simulink model "DUALportRAMinterface_test"  (R2024a)
settings: Solver=FixedStepDiscrete  StartTime=0.0  StopTime=1100  RelTol=1e-3
values from neighbouring files (symbols this model uses):
  Ts = 1/Fs    (= 7.50007500075e-06)    [new_generation_coeff.m]    (also in simon_test.m; simple_fft_test.m = 1/F; testPSD_c2d.m; testPSD_simulink.m)
libraries: hdlsllib x34, simulink x1
settings Model: DataTypeOverride=Off  SimulationMode=rapid-accelerator  Creator=Simon  LastModifiedBy=Simon
settings OptimizationCC: BlockReduction=off  ConditionallyExecuteInputs=off  DefaultParameterBehavior=Inlined  InheritOutputTypeSmallerThanSingle=on
settings DebuggingCC: AlgebraicLoopMsg=error  SingleTaskRateTransMsg=error  UnconnectedInputMsg=warning  UnconnectedOutputMsg=warning  UnconnectedLineMsg=warning
settings HardwareCC: ProdBitPerPointer=32  ProdBitPerSizeT=32  ProdBitPerPtrDiffT=32  ProdLargestAtomicFloat=None  ProdIntDivRoundTo=Undefined  ProdEndianess=Unspecified  ProdWordSize=32  ProdHWDeviceType=ASIC/FPGA->ASIC/FPGA  TargetBitPerPointer=64  TargetBitPerSizeT=64  TargetBitPerPtrDiffT=64  TargetLongLongMode=on  TargetIntDivRoundTo=Zero  TargetEndianess=LittleEndian  TargetWordSize=64  TargetHWDeviceType=Custom Processor->MATLAB Host Computer  ProdEqTarget=off

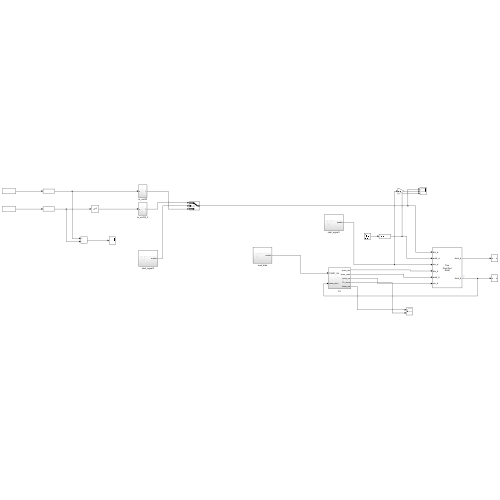
[thumbnail: Simulink's stored preview of the top-level diagram]
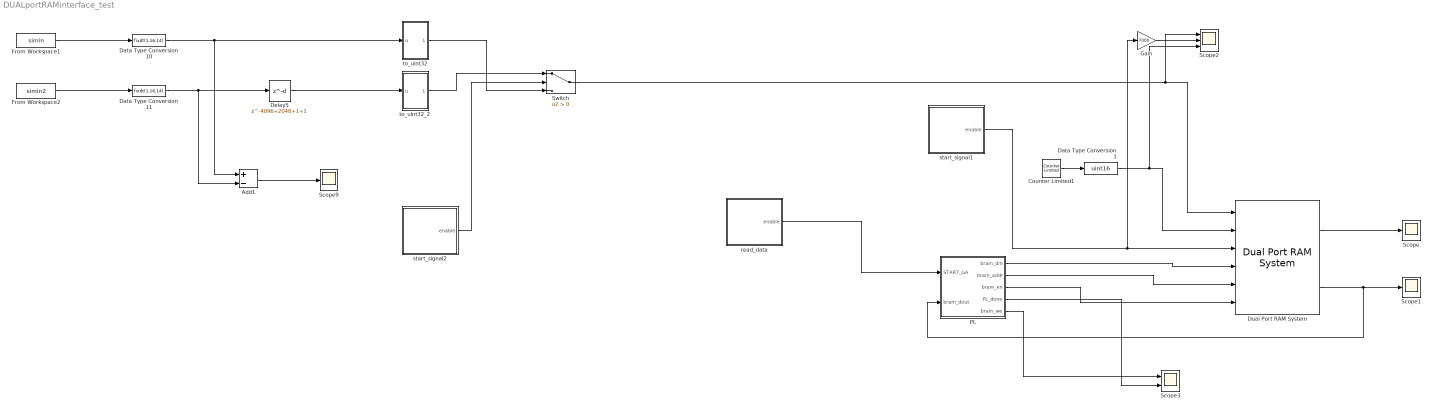
== system DUALportRAMinterface_test ==
  Add1 : Sum  Inputs=+-
  Counter Limited1 : simulink/Sources/Counter Limited  uplimit=14000  tsamp=Ts
  Data Type Conversion1 : DataTypeConversion  OutDataTypeStr=uint16  SaturateOnIntegerOverflow=off  RndMeth=Floor
  Data Type Conversion10 : DataTypeConversion  OutDataTypeStr=fixdt(1,16,14)  SaturateOnIntegerOverflow=off  RndMeth=Floor
  Data Type Conversion11 : DataTypeConversion  OutDataTypeStr=fixdt(1,16,14)  SaturateOnIntegerOverflow=off  RndMeth=Floor
  Delay5 : Delay  DelayLength=4096+2048+1+1  InitialCondition=0  SampleTime=Ts
  Dual Port RAM System : hdlsllib/HDL RAMs/Dual Port RAM System  RAMType=True dual port  AsyncRead=off  WriteOutputValue=New data  RAMInitialValue=0  allowBusInputs=off  WritesHaveOutput=on  NumReads=0  NumWrites=1  SimulateUsing=Code generation
  From Workspace1 : FromWorkspace  VariableName=simin  SampleTime=Ts
  From Workspace2 : FromWorkspace  VariableName=simin2  SampleTime=Ts
  Gain : Gain  Gain=7000
  PL : Subsystem
  Scope : Scope
  Scope1 : Scope
  Scope2 : Scope  NumInputPorts=3
  Scope3 : Scope  NumInputPorts=2
  Scope9 : Scope
  Switch : Switch  Criteria=u2 > Threshold  SaturateOnIntegerOverflow=off  InputSameDT=off  OutDataTypeStr=Inherit: Same as first input
  read_data : Subsystem
  start_signal1 : Subsystem
  start_signal2 : Subsystem
  to_uint32 : Subsystem
  to_uint32_2 : Subsystem
  wires:
  Dual Port RAM System/1 -> Scope/1
  Counter Limited1/1 -> Data Type Conversion1/1
  Data Type Conversion1/1 -> Scope2/3, Dual Port RAM System/2
  start_signal1/1(enable) -> Dual Port RAM System/3, Gain/1
  PL/1(bram_din) -> Dual Port RAM System/4
  PL/2(bram_addr) -> Dual Port RAM System/5
  PL/3(bram_en) -> Dual Port RAM System/6
  Gain/1 -> Scope2/2
  read_data/1(enable) -> PL/1(START_GA)
  Dual Port RAM System/2 -> Scope1/1, PL/2(bram_dout)
  From Workspace1/1 -> Data Type Conversion10/1
  From Workspace2/1 -> Data Type Conversion11/1
  to_uint32/1(Out1) -> Switch/3
  to_uint32_2/1(Out1) -> Switch/1
  start_signal2/1(enable) -> Switch/2
  Delay5/1 -> to_uint32_2/1(u)
  Switch/1 -> Scope2/1, Dual Port RAM System/1
  Data Type Conversion11/1 -> Delay5/1, Add1/2
  Add1/1 -> Scope9/1
  Data Type Conversion10/1 -> Add1/1, to_uint32/1(u)
  PL/4(PL_done) -> Scope3/2
  PL/5(bram_we) -> Scope3/1

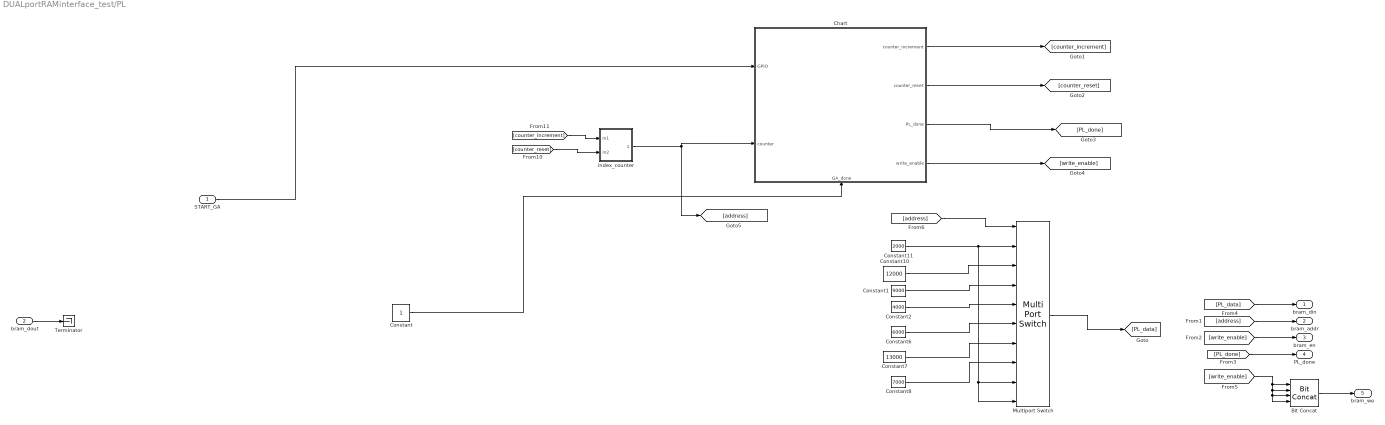
== system DUALportRAMinterface_test/PL ==
  START_GA : Inport
  bram_dout : Inport  Port=2
  Bit Concat : hdlsllib/Logic and Bit Operations/Bit Concat  numInputs=4
  Chart : Stateflow chart  TreatAsAtomicUnit=on
      settings: PortSchema="{\"entries\":[{\"content\":{\"sides\":[{\"content\":{\"connectorIds\":[\"In2\",\"In3\"]},\"type\":\"ConnectorPlacement.EquallySpacedRectSide\",\"uuid\":\"f3ce331f-c708-4668-a9cb-fb327ea74ab5\"},{\"content\":{\"connectorIds\":[\"Out1\",\"Out2\",\"Out3\",\"Out4\"],\"side\":\"RIGHT\"},\"type\":\"ConnectorPlacement.EquallySpacedRectSide\",\"uuid\":\"3766927a-abff-497d-9544-2098881ba174\"},{\"content\":{\"side\":\"TOP\"},\"type\":\"ConnectorPlacement.EquallySpacedRectSide\",\"uuid\":\"ebfe3d64-ee7d-4953-a6ba-e7e40988decf\"},{\"content\":{\"connectorIds\":[\"In1\"],\"side\":\"BOTTOM\"},\"type\":\"ConnectorPlacement.EquallySpacedRectSide\",\"uuid\":\"f39ceaf8-4df7-4e40-9de5-da7597831fb4\"}]},\"type\":\"ConnectorPlacement.EquallySpacedConnector\",\"uuid\":\"89f60450-5933-42bb-b72b-5f8ec55483e0\"}],\"packageUris\":[\"http://schema.mathworks.com/mf0/Connector/R2020b\"],\"version\":\"1.0\"}"
  Constant : Constant  OutDataTypeStr=boolean
  Constant1 : Constant  Value=9000  OutDataTypeStr=uint32  SampleTime=Ts
  Constant10 : Constant  Value=12000  OutDataTypeStr=uint32  SampleTime=Ts
  Constant11 : Constant  Value=2000  OutDataTypeStr=uint32  SampleTime=Ts
  Constant2 : Constant  Value=4000  OutDataTypeStr=uint32  SampleTime=Ts
  Constant6 : Constant  Value=6000  OutDataTypeStr=uint32  SampleTime=Ts
  Constant7 : Constant  Value=13000  OutDataTypeStr=uint32  SampleTime=Ts
  Constant8 : Constant  Value=7000  OutDataTypeStr=uint32  SampleTime=Ts
  Multiport Switch : MultiPortSwitch  DataPortOrder=Specify indices  Inputs=8  DataPortIndices={0,1,2,3,4,5,6,7}  DataPortForDefault=Additional data port  DiagnosticForDefault=None  SaturateOnIntegerOverflow=off  InputSameDT=off
  Terminator : Terminator
  index_counter : Subsystem
  bram_din : Outport
  bram_addr : Outport  Port=2
  bram_en : Outport  Port=3
  PL_done : Outport  Port=4
  bram_we : Outport  Port=5
  wires:
  Multiport Switch/1 -> [PL_data]
  [counter_reset] -> index_counter/2(In2)
  index_counter/1(index_counter) -> Chart/3(counter), [address]
  [address] -> bram_addr/1
  [counter_increment] -> index_counter/1(In1)
  [address] -> Multiport Switch/1
  Chart/4(write_enable) -> [write_enable]
  Constant/1 -> Chart/1(GA_done)
  START_GA/1 -> Chart/2(GPIO)
  Chart/2(counter_reset) -> [counter_reset]
  Chart/1(counter_increment) -> [counter_increment]
  [PL_data] -> bram_din/1
  [write_enable] -> bram_en/1
  Constant11/1 -> Multiport Switch/10, Multiport Switch/9, Multiport Switch/2
  Constant10/1 -> Multiport Switch/3
  Constant1/1 -> Multiport Switch/4
  Constant2/1 -> Multiport Switch/5
  Constant6/1 -> Multiport Switch/6
  Constant7/1 -> Multiport Switch/7
  Constant8/1 -> Multiport Switch/8
  bram_dout/1 -> Terminator/1
  [PL_done] -> PL_done/1
  Chart/3(PL_done) -> [PL_done]
  [write_enable] -> Bit Concat/4, Bit Concat/3, Bit Concat/2, Bit Concat/1
  Bit Concat/1 -> bram_we/1

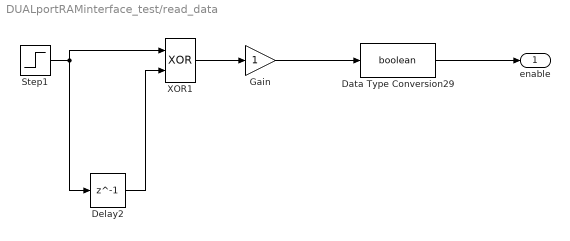
== system DUALportRAMinterface_test/read_data ==
  Data Type Conversion29 : DataTypeConversion  OutDataTypeStr=boolean  SaturateOnIntegerOverflow=off  RndMeth=Floor
  Delay2 : Delay  DelayLength=1  InitialCondition=0  SampleTime=Ts
  Gain : Gain
  Step1 : Step  Time=Ts*14000  SampleTime=Ts
  XOR1 : Logic  Operator=XOR  IconShape=distinctive  AllPortsSameDT=off  OutDataTypeStr=boolean
  enable : Outport
  wires:
  XOR1/1 -> Gain/1
  Step1/1 -> Delay2/1, XOR1/1
  Delay2/1 -> XOR1/2
  Gain/1 -> Data Type Conversion29/1
  Data Type Conversion29/1 -> enable/1

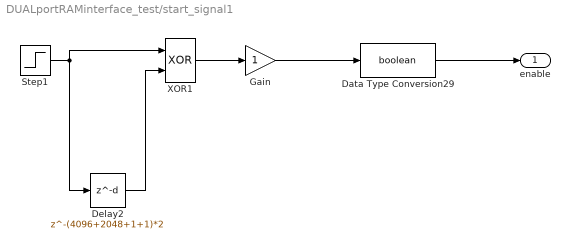
== system DUALportRAMinterface_test/start_signal1 ==
  Data Type Conversion29 : DataTypeConversion  OutDataTypeStr=boolean  SaturateOnIntegerOverflow=off  RndMeth=Floor
  Delay2 : Delay  DelayLength=(4096+2048+1+1)*2  InitialCondition=0  SampleTime=Ts
  Gain : Gain
  Step1 : Step  Time=Ts*0  SampleTime=Ts
  XOR1 : Logic  Operator=XOR  IconShape=distinctive  AllPortsSameDT=off  OutDataTypeStr=boolean
  enable : Outport
  wires:
  Data Type Conversion29/1 -> enable/1
  Gain/1 -> Data Type Conversion29/1
  Delay2/1 -> XOR1/2
  Step1/1 -> XOR1/1, Delay2/1
  XOR1/1 -> Gain/1

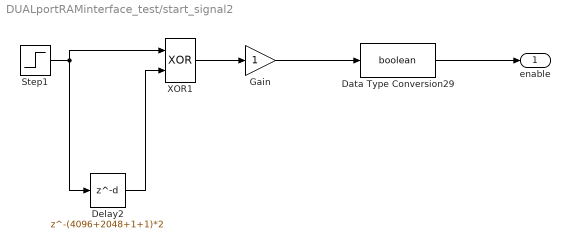
== system DUALportRAMinterface_test/start_signal2 ==
  Data Type Conversion29 : DataTypeConversion  OutDataTypeStr=boolean  SaturateOnIntegerOverflow=off  RndMeth=Floor
  Delay2 : Delay  DelayLength=(4096+2048+1+1)*2  InitialCondition=0  SampleTime=Ts
  Gain : Gain
  Step1 : Step  Time=Ts*(4096+2048+1+1)  SampleTime=Ts
  XOR1 : Logic  Operator=XOR  IconShape=distinctive  AllPortsSameDT=off  OutDataTypeStr=boolean
  enable : Outport
  wires:
  XOR1/1 -> Gain/1
  Step1/1 -> Delay2/1, XOR1/1
  Delay2/1 -> XOR1/2
  Gain/1 -> Data Type Conversion29/1
  Data Type Conversion29/1 -> enable/1

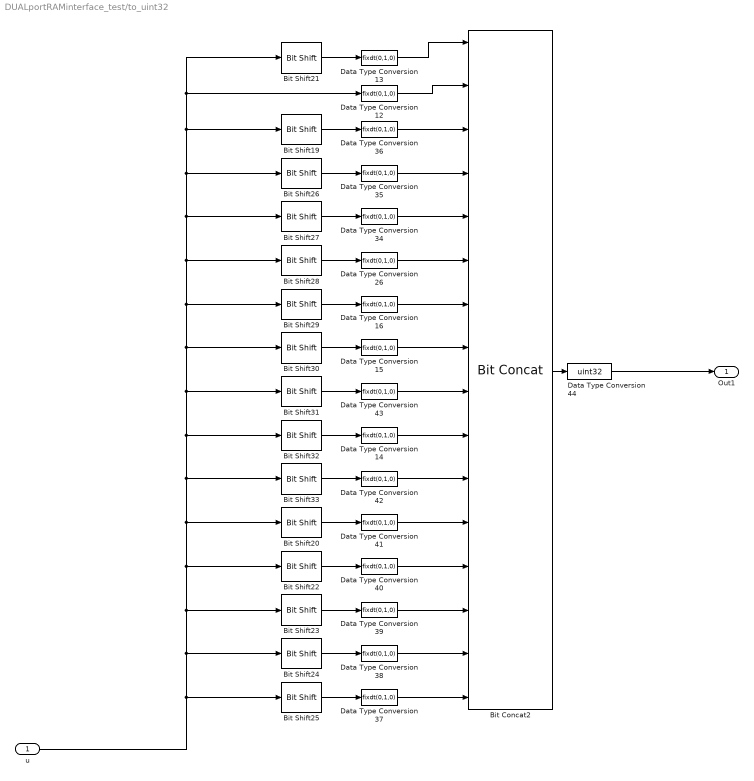
== system DUALportRAMinterface_test/to_uint32 ==
  u : Inport
  Bit Concat2 : hdlsllib/Logic and Bit Operations/Bit Concat  numInputs=16
  Bit Shift19 : hdlsllib/Logic and Bit Operations/Bit Shift  mode=Shift Left Logical  N=1
  Bit Shift20 : hdlsllib/Logic and Bit Operations/Bit Shift  mode=Shift Left Logical  N=10
  Bit Shift21 : hdlsllib/Logic and Bit Operations/Bit Shift  mode=Shift Right Logical  N=1
  Bit Shift22 : hdlsllib/Logic and Bit Operations/Bit Shift  mode=Shift Left Logical  N=11
  Bit Shift23 : hdlsllib/Logic and Bit Operations/Bit Shift  mode=Shift Left Logical  N=12
  Bit Shift24 : hdlsllib/Logic and Bit Operations/Bit Shift  mode=Shift Left Logical  N=13
  Bit Shift25 : hdlsllib/Logic and Bit Operations/Bit Shift  mode=Shift Left Logical  N=14
  Bit Shift26 : hdlsllib/Logic and Bit Operations/Bit Shift  mode=Shift Left Logical  N=2
  Bit Shift27 : hdlsllib/Logic and Bit Operations/Bit Shift  mode=Shift Left Logical  N=3
  Bit Shift28 : hdlsllib/Logic and Bit Operations/Bit Shift  mode=Shift Left Logical  N=4
  Bit Shift29 : hdlsllib/Logic and Bit Operations/Bit Shift  mode=Shift Left Logical  N=5
  Bit Shift30 : hdlsllib/Logic and Bit Operations/Bit Shift  mode=Shift Left Logical  N=6
  Bit Shift31 : hdlsllib/Logic and Bit Operations/Bit Shift  mode=Shift Left Logical  N=7
  Bit Shift32 : hdlsllib/Logic and Bit Operations/Bit Shift  mode=Shift Left Logical  N=8
  Bit Shift33 : hdlsllib/Logic and Bit Operations/Bit Shift  mode=Shift Left Logical  N=9
  Data Type Conversion{12..16,26,34..43} (16 alike) : DataTypeConversion  OutDataTypeStr=fixdt(0,1,0)  SaturateOnIntegerOverflow=off  RndMeth=Floor
  Data Type Conversion44 : DataTypeConversion  OutDataTypeStr=uint32  SaturateOnIntegerOverflow=off  RndMeth=Floor
  Out1 : Outport
  wires:
  Bit Shift22/1 -> Data Type Conversion40/1
  Bit Shift27/1 -> Data Type Conversion34/1
  Data Type Conversion36/1 -> Bit Concat2/3
  u/1 -> Bit Shift21/1, Data Type Conversion12/1, Bit Shift19/1, Bit Shift26/1, Bit Shift27/1, Bit Shift28/1, Bit Shift29/1, Bit Shift30/1, Bit Shift31/1, Bit Shift32/1, Bit Shift33/1, Bit Shift20/1, Bit Shift22/1, Bit Shift23/1, Bit Shift24/1, Bit Shift25/1
  Bit Shift20/1 -> Data Type Conversion41/1
  Data Type Conversion13/1 -> Bit Concat2/1
  Data Type Conversion40/1 -> Bit Concat2/13
  Bit Shift31/1 -> Data Type Conversion43/1
  Data Type Conversion26/1 -> Bit Concat2/6
  Data Type Conversion44/1 -> Out1/1
  Data Type Conversion35/1 -> Bit Concat2/4
  Data Type Conversion42/1 -> Bit Concat2/11
  Bit Shift19/1 -> Data Type Conversion36/1
  Data Type Conversion38/1 -> Bit Concat2/15
  Bit Shift25/1 -> Data Type Conversion37/1
  Data Type Conversion15/1 -> Bit Concat2/8
  Bit Shift30/1 -> Data Type Conversion15/1
  Data Type Conversion12/1 -> Bit Concat2/2
  Bit Shift32/1 -> Data Type Conversion14/1
  Data Type Conversion39/1 -> Bit Concat2/14
  Data Type Conversion34/1 -> Bit Concat2/5
  Data Type Conversion43/1 -> Bit Concat2/9
  Data Type Conversion16/1 -> Bit Concat2/7
  Bit Shift33/1 -> Data Type Conversion42/1
  Bit Shift24/1 -> Data Type Conversion38/1
  Data Type Conversion41/1 -> Bit Concat2/12
  Bit Shift23/1 -> Data Type Conversion39/1
  Bit Shift29/1 -> Data Type Conversion16/1
  Data Type Conversion37/1 -> Bit Concat2/16
  Bit Shift28/1 -> Data Type Conversion26/1
  Bit Shift21/1 -> Data Type Conversion13/1
  Bit Shift26/1 -> Data Type Conversion35/1
  Bit Concat2/1 -> Data Type Conversion44/1
  Data Type Conversion14/1 -> Bit Concat2/10

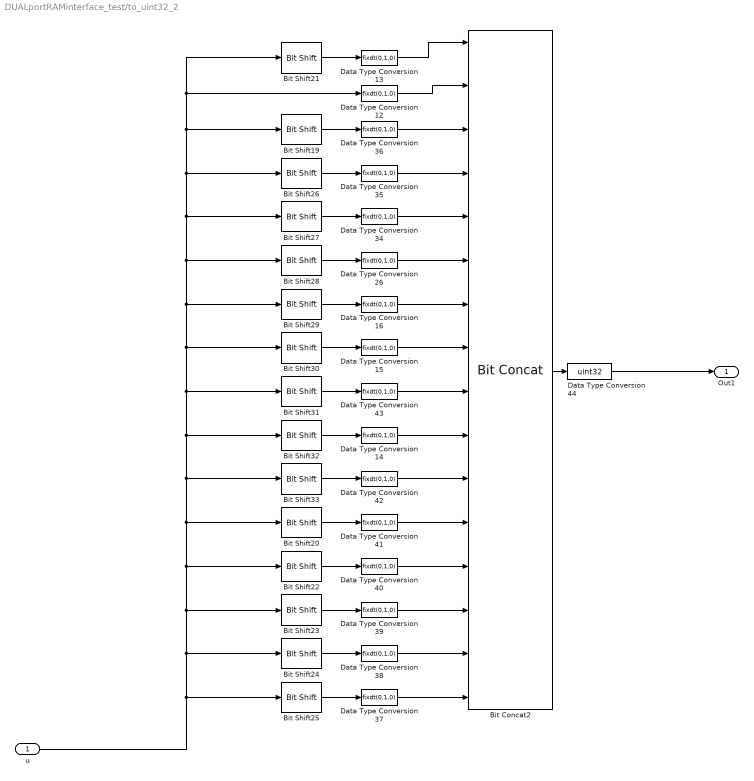
== system DUALportRAMinterface_test/to_uint32_2 ==
  u : Inport
  Bit Concat2 : hdlsllib/Logic and Bit Operations/Bit Concat  numInputs=16
  Bit Shift19 : hdlsllib/Logic and Bit Operations/Bit Shift  mode=Shift Left Logical  N=1
  Bit Shift20 : hdlsllib/Logic and Bit Operations/Bit Shift  mode=Shift Left Logical  N=10
  Bit Shift21 : hdlsllib/Logic and Bit Operations/Bit Shift  mode=Shift Right Logical  N=1
  Bit Shift22 : hdlsllib/Logic and Bit Operations/Bit Shift  mode=Shift Left Logical  N=11
  Bit Shift23 : hdlsllib/Logic and Bit Operations/Bit Shift  mode=Shift Left Logical  N=12
  Bit Shift24 : hdlsllib/Logic and Bit Operations/Bit Shift  mode=Shift Left Logical  N=13
  Bit Shift25 : hdlsllib/Logic and Bit Operations/Bit Shift  mode=Shift Left Logical  N=14
  Bit Shift26 : hdlsllib/Logic and Bit Operations/Bit Shift  mode=Shift Left Logical  N=2
  Bit Shift27 : hdlsllib/Logic and Bit Operations/Bit Shift  mode=Shift Left Logical  N=3
  Bit Shift28 : hdlsllib/Logic and Bit Operations/Bit Shift  mode=Shift Left Logical  N=4
  Bit Shift29 : hdlsllib/Logic and Bit Operations/Bit Shift  mode=Shift Left Logical  N=5
  Bit Shift30 : hdlsllib/Logic and Bit Operations/Bit Shift  mode=Shift Left Logical  N=6
  Bit Shift31 : hdlsllib/Logic and Bit Operations/Bit Shift  mode=Shift Left Logical  N=7
  Bit Shift32 : hdlsllib/Logic and Bit Operations/Bit Shift  mode=Shift Left Logical  N=8
  Bit Shift33 : hdlsllib/Logic and Bit Operations/Bit Shift  mode=Shift Left Logical  N=9
  Data Type Conversion{12..16,26,34..43} (16 alike) : DataTypeConversion  OutDataTypeStr=fixdt(0,1,0)  SaturateOnIntegerOverflow=off  RndMeth=Floor
  Data Type Conversion44 : DataTypeConversion  OutDataTypeStr=uint32  SaturateOnIntegerOverflow=off  RndMeth=Floor
  Out1 : Outport
  wires:
  Data Type Conversion14/1 -> Bit Concat2/10
  Bit Concat2/1 -> Data Type Conversion44/1
  Bit Shift26/1 -> Data Type Conversion35/1
  Bit Shift21/1 -> Data Type Conversion13/1
  Bit Shift28/1 -> Data Type Conversion26/1
  Data Type Conversion37/1 -> Bit Concat2/16
  Bit Shift29/1 -> Data Type Conversion16/1
  Bit Shift23/1 -> Data Type Conversion39/1
  Data Type Conversion41/1 -> Bit Concat2/12
  Bit Shift24/1 -> Data Type Conversion38/1
  Bit Shift33/1 -> Data Type Conversion42/1
  Data Type Conversion16/1 -> Bit Concat2/7
  Data Type Conversion43/1 -> Bit Concat2/9
  Data Type Conversion34/1 -> Bit Concat2/5
  Data Type Conversion39/1 -> Bit Concat2/14
  Bit Shift32/1 -> Data Type Conversion14/1
  Data Type Conversion12/1 -> Bit Concat2/2
  Bit Shift30/1 -> Data Type Conversion15/1
  Data Type Conversion15/1 -> Bit Concat2/8
  Bit Shift25/1 -> Data Type Conversion37/1
  Data Type Conversion38/1 -> Bit Concat2/15
  Bit Shift19/1 -> Data Type Conversion36/1
  Data Type Conversion42/1 -> Bit Concat2/11
  Data Type Conversion35/1 -> Bit Concat2/4
  Data Type Conversion44/1 -> Out1/1
  Data Type Conversion26/1 -> Bit Concat2/6
  Bit Shift31/1 -> Data Type Conversion43/1
  Data Type Conversion40/1 -> Bit Concat2/13
  Data Type Conversion13/1 -> Bit Concat2/1
  Bit Shift20/1 -> Data Type Conversion41/1
  u/1 -> Bit Shift25/1, Bit Shift24/1, Bit Shift23/1, Bit Shift22/1, Bit Shift20/1, Bit Shift33/1, Bit Shift32/1, Bit Shift31/1, Bit Shift30/1, Bit Shift29/1, Bit Shift28/1, Bit Shift27/1, Bit Shift26/1, Bit Shift19/1, Data Type Conversion12/1, Bit Shift21/1
  Data Type Conversion36/1 -> Bit Concat2/3
  Bit Shift27/1 -> Data Type Conversion34/1
  Bit Shift22/1 -> Data Type Conversion40/1

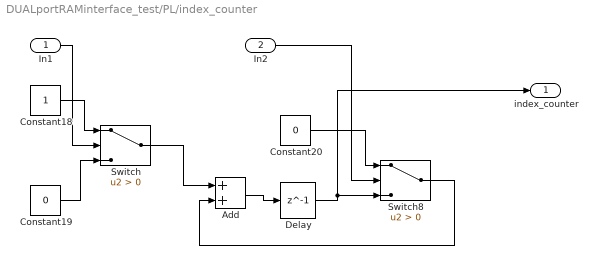
== system DUALportRAMinterface_test/PL/index_counter ==
  In1 : Inport
  In2 : Inport  Port=2
  Add : Sum  OutDataTypeStr=Inherit: Same as first input
  Constant18 : Constant  OutDataTypeStr=fixdt(0,16,0)  SampleTime=Ts
  Constant19 : Constant  Value=0  OutDataTypeStr=fixdt(0,16,0)  SampleTime=Ts
  Constant20 : Constant  Value=0  OutDataTypeStr=uint16  SampleTime=Ts
  Delay : Delay  DelayLength=1  InitialCondition=0  SampleTime=Ts
  Switch : Switch  Criteria=u2 > Threshold  SaturateOnIntegerOverflow=off  InputSameDT=off  OutDataTypeStr=Inherit: Same as first input
  Switch8 : Switch  Criteria=u2 > Threshold  SaturateOnIntegerOverflow=off  InputSameDT=off  OutDataTypeStr=Inherit: Same as first input
  index_counter : Outport
  wires:
  Constant19/1 -> Switch/3
  Switch8/1 -> Add/2
  Switch/1 -> Add/1
  Delay/1 -> index_counter/1, Switch8/3
  In2/1 -> Switch8/2
  Add/1 -> Delay/1
  Constant20/1 -> Switch8/1
  Constant18/1 -> Switch/1
  In1/1 -> Switch/2

== stateflow chart DUALportRAMinterface_test/PL/Chart ==
  settings: executeAtInitialization=1
  state initial_wait_state
    entry:
    counter_increment = false;
    counter_reset = true;
    write_enable = false;
    PL_done = false;
  state PL_read_data
    entry:
    counter_increment = true;
    counter_reset = false;
    write_enable = false;
    PL_done = false;
  state wait_for_GA_done
    entry:
    counter_increment = false;
    counter_reset = true;
    write_enable = false;
    PL_done = false;
  state reset_state
    entry:
    counter_increment = false;
    counter_reset = true;
    write_enable = false;
    PL_done = true;
  state PL_write_data_back
    entry:
    counter_increment = true;
    counter_reset = false;
    write_enable = true;
    PL_done = false;
  (default) -> initial_wait_state
  initial_wait_state -> PL_read_data : [GPIO == 1]
  PL_read_data -> wait_for_GA_done : [counter == (4096+2048+1)*2]
  wait_for_GA_done -> PL_write_data_back : [GA_done == 1]
  PL_write_data_back -> reset_state : [counter == 8]
  data: GA_done input boolean; GPIO input; counter input; counter_increment output boolean; counter_reset output boolean; PL_done output boolean; write_enable output boolean
